simulink model "Simulink_6DoF_RV"  (R2021b)
settings: Solver=ode4  StartTime=0.0  StopTime=T_run  FixedStep=0.01  RelTol=1e-3
values from neighbouring files (symbols this model uses):
  alpha = 5    [MAIN_6DoF_RV.m]    (also in Simulatore_script_gruppo6.m)
  beta = 10    [MAIN_6DoF_RV.m]    (also in Simulatore_script_gruppo6.m)
  control = 2    [MAIN_6DoF_RV.m]    (also in Simulatore_script_gruppo6.m)
  den_pos = [Tm_pos 1]    [MAIN_6DoF_RV.m]    (also in Simulatore_script_gruppo6.m)
  dt_Fx1_PH1 = (1+dtx_PH1_corr)*dt_Fx1_PH1id    (= 48.314973357)    [MAIN_6DoF_RV.m]    (also in Simulatore_script_gruppo6.m)
  Dt_var = 0.1    [MAIN_6DoF_RV.m]    (also in Simulatore_script_gruppo6.m)
  dtz_PH2_corr = 0.28    [MAIN_6DoF_RV.m]    (also in Simulatore_script_gruppo6.m)
  epsilon = 1e-3    (= 0.001)    [MAIN_6DoF_RV.m]    (also in Simulatore_script_gruppo6.m)
  epsilon_FA = 0.005    [MAIN_6DoF_RV.m]    (also in Simulatore_script_gruppo6.m)
  F_D = 1/2*rho*CD*A*vc^2    [MAIN_6DoF_RV.m]    (also in Simulatore_script_gruppo6.m)
  fa_control = 2    [MAIN_6DoF_RV.m]    (also in Simulatore_script_gruppo6.m)
  FJ2_r4 = -mc*(3*J2*mu*r_E^2)/2    (= -1.15338103268e+24)    [MAIN_6DoF_RV.m]    (also in Simulatore_script_gruppo6.m)
  Fx_PH1id = Tmax    (= 1)    [MAIN_6DoF_RV.m]    (also in Simulatore_script_gruppo6.m)
  Fz_PH2id = Tmax    (= 1)    [MAIN_6DoF_RV.m]    (also in Simulatore_script_gruppo6.m)
  I = [Jx  0   0 ... (first row only)    [MAIN_6DoF_RV.m]    (also in Simulatore_script_gruppo6.m)
  Id = eye(3)    [MAIN_6DoF_RV.m]    (also in Simulatore_script_gruppo6.m)
  invI = inv(I)    [MAIN_6DoF_RV.m]    (also in Simulatore_script_gruppo6.m)
  K_d = diag([d1,d2,d3])    [MAIN_6DoF_RV.m]    (also in Simulatore_script_gruppo6.m)
  lambda = 0.06    [MAIN_6DoF_RV.m]    (also in Simulatore_script_gruppo6.m)
  lambda_FA = 0.07    [MAIN_6DoF_RV.m]    (also in Simulatore_script_gruppo6.m)
  mc = 43.8    [MAIN_6DoF_RV.m]    (also in Simulatore_script_gruppo6.m)
  mu = 3.986012*10^14    (= 398601200000000)    [MAIN_6DoF_RV.m]    (also in Simulatore_script_gruppo6.m)
  num_pos = Km_pos    (= 4)    [MAIN_6DoF_RV.m]    (also in Simulatore_script_gruppo6.m)
  omega = (mu/r_t^3)^0.5    (= 0.00113136572666)    [MAIN_6DoF_RV.m]    (also in Simulatore_script_gruppo6.m)
  omega_0 = [0 0 0]    [MAIN_6DoF_RV.m]    (also in Simulatore_script_gruppo6.m)
  q0_0 = 0.5    [MAIN_6DoF_RV.m]    (also in Simulatore_script_gruppo6.m)
  q0_des = quat0_PH3(1)    [MAIN_6DoF_RV.m]    (also in Simulatore_script_gruppo6.m)
  qv_0 = [0.5 0.5 0.5]    [MAIN_6DoF_RV.m]    (also in Simulatore_script_gruppo6.m)
  r0 = [Xo Yo Zo]    [MAIN_6DoF_RV.m]    (also in Simulatore_script_gruppo6.m)
  r0_p1Id = [x0_PH1, y0_PH1, z0_PH1]    [MAIN_6DoF_RV.m]    (also in Simulatore_script_gruppo6.m)
  r0_p3Id = [x0_PH3 y0_PH3 z0_PH3]    [MAIN_6DoF_RV.m]    (also in Simulatore_script_gruppo6.m)
  r_des_fa = [xf yf zf]    [MAIN_6DoF_RV.m]    (also in Simulatore_script_gruppo6.m)
  r_t = r_E + height    (= 6778145)    [MAIN_6DoF_RV.m]    (also in Simulatore_script_gruppo6.m)
  t_acc_fa = (1+dtx_PH3_corr)*t_acc_fa_id    [MAIN_6DoF_RV.m]    (also in Simulatore_script_gruppo6.m)
  tau_RW = 0.25    [MAIN_6DoF_RV.m]    (also in Simulatore_script_gruppo6.m)
  Tmax = n*Fthr    (= 1)    [MAIN_6DoF_RV.m]    (also in Simulatore_script_gruppo6.m)
  U_max = 0.25    [MAIN_6DoF_RV.m]    (also in Simulatore_script_gruppo6.m)
  U_max_RW = 1e-3    (= 0.001)    [MAIN_6DoF_RV.m]    (also in Simulatore_script_gruppo6.m)
  U_off_pos = 0.60*U_on_pos    (= 0.6)    [MAIN_6DoF_RV.m]    (also in Simulatore_script_gruppo6.m)
  U_on_pos = 1    [MAIN_6DoF_RV.m]    (also in Simulatore_script_gruppo6.m)
  v0 = [Vxo Vyo Vzo]    [MAIN_6DoF_RV.m]    (also in Simulatore_script_gruppo6.m)
  v_des_fa = [vxf vyf vzf]    [MAIN_6DoF_RV.m]    (also in Simulatore_script_gruppo6.m)
  Vx_max = 0.15    [MAIN_6DoF_RV.m]    (also in Simulatore_script_gruppo6.m)
  x0_PH2 = -3000    [MAIN_6DoF_RV.m]    (also in Simulatore_script_gruppo6.m)
  x0_PH3 = -500    [MAIN_6DoF_RV.m]    (also in Simulatore_script_gruppo6.m)
  x_start_dec = r_des_fa(1)-(v_des_fa(1)^2-(Vx_max*(1+dtx_PH3_corr))^2)/(2*(Fx_dec/mc))    [MAIN_6DoF_RV.m]    (also in Simulatore_script_gruppo6.m)
  xf = -2    [MAIN_6DoF_RV.m]    (also in Simulatore_script_gruppo6.m)
  Z0_RW = [sqrt(3)/2    0           -sqrt(3)/2  0 ... (first row only)    [MAIN_6DoF_RV.m]    (also in Simulatore_script_gruppo6.m)
  z_start_Fx2_PH1id = 0.5*(DVx2*(1+dtx_PH1_corr))^2/(Fx_PH1id/mc)    (= 26.6476786585)    [MAIN_6DoF_RV.m]    (also in Simulatore_script_gruppo6.m)
  z_start_Fz2_PH2id = 0.5*(DVz2*(1+dtz_PH2_corr))^2/(Fz_PH2id/mc)    [MAIN_6DoF_RV.m]    (also in Simulatore_script_gruppo6.m)
  Zinv = pinv(Z0_RW)    [MAIN_6DoF_RV.m]    (also in Simulatore_script_gruppo6.m)
libraries: vrlib x3, robotcorelib x1
(part 1 of 2)
settings Model: SimulationMode=rapid-accelerator  Creator=Asus  LastModifiedBy=Asus
settings SolverCC: AlgebraicLoopSolver=TrustRegion
settings DebuggingCC: ArithmeticOperatorsInVariantConditions=warning
settings SFSimCC: CustomCodeUndefinedFunction=UseInterfaceOnly

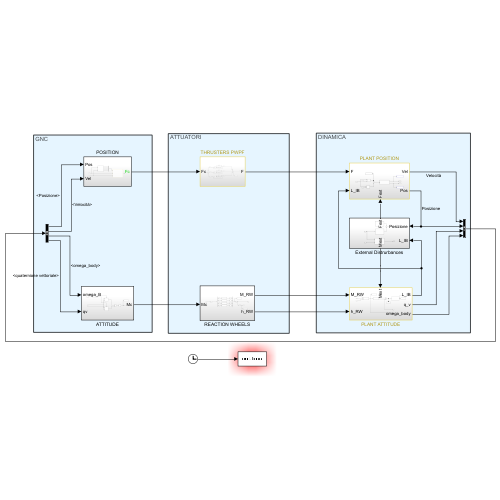
[thumbnail: Simulink's stored preview of the top-level diagram]
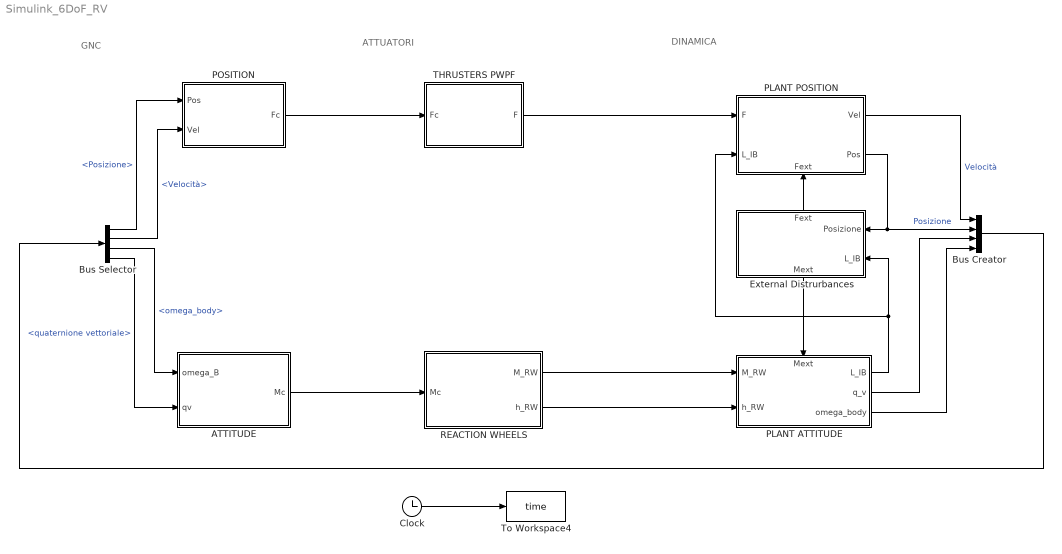
== system Simulink_6DoF_RV ==
  note: DINAMICA
  note: ATTUATORI
  note: GNC
  ATTITUDE : Subsystem  SystemSampleTime=0.02
  Bus Creator : BusCreator  Inputs=4
  Bus Selector : BusSelector  OutputSignals=Posizione,Velocità,omega_body,quaternione vettoriale
  Clock : Clock
  External Distrurbances : Subsystem
      settings: PortSchema="{\"entries\":[{\"content\":{\"sides\":[{\"content\":{\"connectorIds\":[]},\"type\":\"ConnectorPlacement.EquallySpacedRectSide\",\"uuid\":\"40a47393-8969-4a4a-bb19-fe76317a4dc1\"},{\"content\":{\"connectorIds\":[\"In1\",\"In2\"],\"side\":\"RIGHT\"},\"type\":\"ConnectorPlacement.EquallySpacedRectSide\",\"uuid\":\"517d6888-1d4e-40fb-9a61-dcbe45465223\"},{\"content\":{\"connectorIds\":[\"Out2\"],\"side\":\"TOP\"},\"type\":\"ConnectorPlacement.EquallySpacedRectSide\",\"uuid\":\"885891b7-149a-48f0-ba9b-916a7b55094e\"},{\"content\":{\"connectorIds\":[\"Out1\"],\"side\":\"BOTTOM\"},\"type\":\"ConnectorPlacement.EquallySpacedRectSide\",\"uuid\":\"c8000deb-5487-4091-9eab-42d91257081e\"}]},\"type\":\"ConnectorPlacement.EquallySpacedConnector\",\"uuid\":\"af16e5ba-db8c-4edd-a4d6-30205250b632\"}],\"packageUris\":[\"http://schema.mathworks.com/mf0/Connector/R2020b\"],\"version\":\"1.0\"}"
  PLANT ATTITUDE : Subsystem
      settings: PortSchema="{\"entries\":[{\"content\":{\"sides\":[{\"content\":{\"connectorIds\":[\"In1\",\"In2\"]},\"type\":\"ConnectorPlacement.EquallySpacedRectSide\",\"uuid\":\"5bd07662-f93f-4a51-a4b7-c766d18c6c52\"},{\"content\":{\"connectorIds\":[\"Out1\",\"Out2\",\"Out3\"],\"side\":\"RIGHT\"},\"type\":\"ConnectorPlacement.EquallySpacedRectSide\",\"uuid\":\"400ce1e4-a5e5-4d4b-bb84-f2deb9eca011\"},{\"content\":{\"connectorIds\":[\"In3\"],\"side\":\"TOP\"},\"type\":\"ConnectorPlacement.EquallySpacedRectSide\",\"uuid\":\"a16ccc55-2fa1-4b33-bfe9-424ec0136aee\"}]},\"type\":\"ConnectorPlacement.EquallySpacedConnector\",\"uuid\":\"0051f69f-69f8-4575-b5c3-4b5124977914\"}],\"packageUris\":[\"http://schema.mathworks.com/mf0/Connector/R2020b\"],\"version\":\"1.0\"}"
  PLANT POSITION : Subsystem
      settings: PortSchema="{\"entries\":[{\"content\":{\"sides\":[{\"content\":{\"connectorIds\":[\"In1\",\"In2\"]},\"type\":\"ConnectorPlacement.EquallySpacedRectSide\",\"uuid\":\"6f851545-3e44-41e1-9040-e1da3530ae0f\"},{\"content\":{\"connectorIds\":[\"Out1\",\"Out2\"],\"side\":\"RIGHT\"},\"type\":\"ConnectorPlacement.EquallySpacedRectSide\",\"uuid\":\"a0bf2e2b-c069-45ff-9cba-5c6c5f5dd88c\"},{\"content\":{\"connectorIds\":[],\"side\":\"TOP\"},\"type\":\"ConnectorPlacement.EquallySpacedRectSide\",\"uuid\":\"79f05063-7ba4-40b0-bcbd-aeb89fa83470\"},{\"content\":{\"connectorIds\":[\"In3\"],\"side\":\"BOTTOM\"},\"type\":\"ConnectorPlacement.EquallySpacedRectSide\",\"uuid\":\"12fcf113-d807-4585-8c70-f8ca37fce548\"}]},\"type\":\"ConnectorPlacement.EquallySpacedConnector\",\"uuid\":\"de90291e-fe15-4172-840f-0b421646e685\"}],\"packageUris\":[\"http://schema.mathworks.com/mf0/Connector/R2020b\"],\"version\":\"1.0\"}"
  POSITION : Subsystem  SystemSampleTime=0.01
      settings: MinAlgLoopOccurrences=on
  REACTION WHEELS : Subsystem
  THRUSTERS PWPF : Subsystem
  To Workspace4 : ToWorkspace  VariableName=time  SampleTime=Dt_var
  wires:
  Clock/1 -> To Workspace4/1
  PLANT POSITION/2(Pos) -> External Distrurbances/1(Posizione), Bus Creator/2  "Posizione"
  PLANT POSITION/1(Vel) -> Bus Creator/1  "Velocità"
  REACTION WHEELS/2(h_RW) -> PLANT ATTITUDE/2(h_RW)
  REACTION WHEELS/1(M_RW) -> PLANT ATTITUDE/1(M_RW)
  PLANT ATTITUDE/2(q_v) -> Bus Creator/3
  PLANT ATTITUDE/3(omega_body) -> Bus Creator/4
  ATTITUDE/1(Mc) -> REACTION WHEELS/1(Mc)
  Bus Selector/3 -> ATTITUDE/1(omega_B)  "<omega_body>"
  Bus Selector/4 -> ATTITUDE/2(qv)  "<quaternione vettoriale>"
  PLANT ATTITUDE/1(L_IB) -> External Distrurbances/2(L_IB), PLANT POSITION/2(L_IB)
  Bus Selector/1 -> POSITION/1(Pos)  "<Posizione>"
  Bus Selector/2 -> POSITION/2(Vel)  "<Velocità>"
  External Distrurbances/1(Mext) -> PLANT ATTITUDE/3(Mext)
  POSITION/1(Fc) -> THRUSTERS PWPF/1(Fc)
  Bus Creator/1 -> Bus Selector/1
  THRUSTERS PWPF/1(F) -> PLANT POSITION/1(F)
  External Distrurbances/2(Fext) -> PLANT POSITION/3(Fext)

== system Simulink_6DoF_RV/ATTITUDE ==
  omega_B : Inport
  qv : Inport  Port=2
  Constant : Constant  Value=control
  Merge : Merge
  PD 4 : Subsystem  TreatAsAtomicUnit=on
  Rate Transition : RateTransition  OutPortSampleTime=0.02
  SMC : Subsystem  TreatAsAtomicUnit=on
  Switch Case : SwitchCase  CaseConditions={2,1}  ShowDefaultCase=off
  To Workspace2 : ToWorkspace  VariableName=Mc  SampleTime=Dt_var
  Mc : Outport
  wires:
  Merge/1 -> Rate Transition/1
  Switch Case/2 -> PD 4/Action
  PD 4/1(Mc) -> Merge/2
  Constant/1 -> Switch Case/1
  omega_B/1 -> SMC/1("omega_B "), PD 4/1(omega_B)  "omega_body"
  SMC/1(Mc) -> Merge/1
  Switch Case/1 -> SMC/Action
  qv/1 -> PD 4/2(qv), SMC/2(qv)  "quaternione vettoriale"
  Rate Transition/1 -> To Workspace2/1, Mc/1

== system Simulink_6DoF_RV/External Distrurbances ==
  Posizione : Inport
  L_IB : Inport  Port=2
  Drag : Subsystem
  Gravity Gradient : Subsystem
  J2 : Subsystem
  Sum : Sum
  Mext : Outport
  Fext : Outport  Port=2
  wires:
  Drag/1(Fa) -> Sum/1
  Sum/1 -> Fext/1
  J2/1(Fj2) -> Sum/2
  Gravity Gradient/1(Mgg) -> Mext/1
  Posizione/1 -> Gravity Gradient/1(Posizione1), J2/1(Posizione)
  L_IB/1 -> Gravity Gradient/2(L_IB)

== system Simulink_6DoF_RV/PLANT ATTITUDE ==
  M_RW : Inport
  h_RW : Inport  Port=2
  Mext : Inport  Port=3
  Coordinate Transformation Conversion : robotcorelib/Coordinate Transformation Conversion  InputRepresentation=Quaternion  InputEulerSequence=ZYX  ShowTrVecInputPort=on  OutputRepresentation=Rotation Matrix  OutputEulerSequence=ZYX  ShowTrVecOutputPort=on  SimulateUsing=Interpreted execution
      settings: SourceProductBaseCode=NV,RO,RR,UV
  Eq. eulero : Subsystem
  Mux : Mux  Inputs=2
  To Workspace : ToWorkspace  VariableName=omega_B  SampleTime=Dt_var
  To Workspace1 : ToWorkspace  VariableName=q  SampleTime=Dt_var
  To Workspace5 : ToWorkspace  VariableName=L  SampleTime=Dt_var
  quaternioni : Subsystem
  L_IB : Outport
  q_v : Outport  Port=2
  omega_body : Outport  Port=3
  wires:
  quaternioni/1(q0) -> Mux/1
  Eq. eulero/1(omega_B) -> To Workspace/1, omega_body/1, quaternioni/1(omega_B)  "omega_body"
  Mux/1 -> Coordinate Transformation Conversion/1, To Workspace1/1
  M_RW/1 -> Eq. eulero/3(M_RW)
  h_RW/1 -> Eq. eulero/2(h_RW)
  Coordinate Transformation Conversion/1 -> L_IB/1, To Workspace5/1
  quaternioni/2(qv) -> q_v/1, Mux/2  "quaternione vettoriale"
  Mext/1 -> Eq. eulero/1(M)

== system Simulink_6DoF_RV/PLANT POSITION ==
  F : Inport
  L_IB : Inport  Port=2
  Fext : Inport  Port=3
  HILL eqs : Subsystem
  Matrix Multiply : Product  Multiplication=Matrix(*)
  Matrix Multiply1 : Product  Multiplication=Matrix(*)
  Sum3 : Sum
  To Workspace1 : ToWorkspace  VariableName=Pos  SampleTime=Dt_var
  To Workspace2 : ToWorkspace  VariableName=Vel  SampleTime=Dt_var
  To Workspace3 : ToWorkspace  VariableName=F_LVLH  SampleTime=Dt_var
  Vel : Outport
  Pos : Outport  Port=2
  wires:
  F/1 -> Matrix Multiply1/2
  L_IB/1 -> Matrix Multiply/1, Matrix Multiply1/1
  Matrix Multiply1/1 -> To Workspace3/1, Sum3/1
  Matrix Multiply/1 -> Sum3/2
  Fext/1 -> Matrix Multiply/2
  HILL eqs/2(Out2) -> To Workspace2/1, Vel/1
  Sum3/1 -> HILL eqs/1(In1)
  HILL eqs/1(Pos) -> To Workspace1/1, Pos/1

== system Simulink_6DoF_RV/POSITION ==
  Pos : Inport
  Vel : Inport  Port=2
  Bus Creator : BusCreator  Inputs=5
  Maneuvers : Subsystem
  Position and Guidance : Subsystem
  Fc : Outport
  wires:
  Vel/1 -> Position and Guidance/3(Vel), Maneuvers/2(Vel)
  Pos/1 -> Position and Guidance/2(Pos), Maneuvers/1(Pos)
  Position and Guidance/1(Fc) -> Fc/1
  Maneuvers/1(Phase number) -> Bus Creator/1  "phase number"
  Maneuvers/2(off_PH1.1) -> Bus Creator/2  "off_PH1:1"
  Maneuvers/3(off_PH1.2) -> Bus Creator/3  "off_PH1:2"
  Maneuvers/4(off_PH2.1) -> Bus Creator/4  "off_PH2:1"
  Maneuvers/5(off_PH2.2) -> Bus Creator/5  "off_PH2:2"
  Bus Creator/1 -> Position and Guidance/1(Phase)

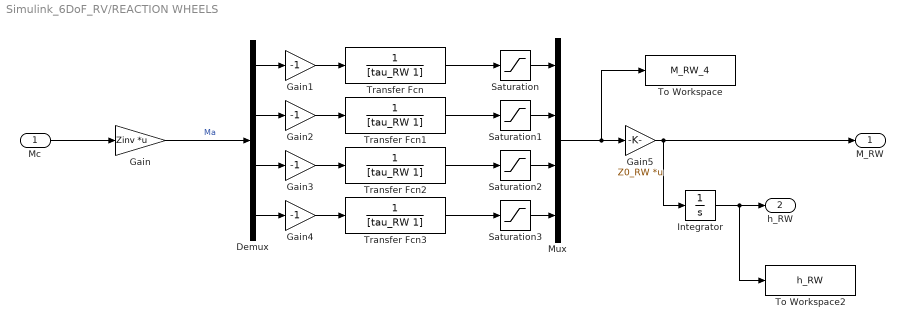
== system Simulink_6DoF_RV/REACTION WHEELS ==
  Mc : Inport
  Demux : Demux
  Gain : Gain  Gain=Zinv  Multiplication=Matrix(K*u)
  Gain{1..4} (4 alike) : Gain  Gain=-1
  Gain5 : Gain  Gain=Z0_RW  Multiplication=Matrix(K*u)
  Integrator : Integrator
  Mux : Mux
  Saturation{,1..3} (4 alike) : Saturate  UpperLimit=U_max_RW  LowerLimit=-U_max_RW
  To Workspace : ToWorkspace  VariableName=M_RW_4  SampleTime=Dt_var
  To Workspace2 : ToWorkspace  VariableName=h_RW  SampleTime=Dt_var
  Transfer Fcn{,1..3} (4 alike) : TransferFcn  Denominator=[tau_RW 1]
  M_RW : Outport
  h_RW : Outport  Port=2
  wires:
  Demux/4 -> Gain4/1
  Mc/1 -> Gain/1
  Demux/1 -> Gain1/1
  Transfer Fcn2/1 -> Saturation2/1
  Gain3/1 -> Transfer Fcn2/1
  Gain/1 -> Demux/1  "Ma"
  Saturation/1 -> Mux/1
  Gain5/1 -> M_RW/1, Integrator/1
  Gain4/1 -> Transfer Fcn3/1
  Transfer Fcn3/1 -> Saturation3/1
  Saturation3/1 -> Mux/4
  Transfer Fcn1/1 -> Saturation1/1
  Gain2/1 -> Transfer Fcn1/1
  Transfer Fcn/1 -> Saturation/1
  Saturation2/1 -> Mux/3
  Demux/3 -> Gain3/1
  Gain1/1 -> Transfer Fcn/1
  Integrator/1 -> To Workspace2/1, h_RW/1
  Mux/1 -> To Workspace/1, Gain5/1
  Demux/2 -> Gain2/1
  Saturation1/1 -> Mux/2

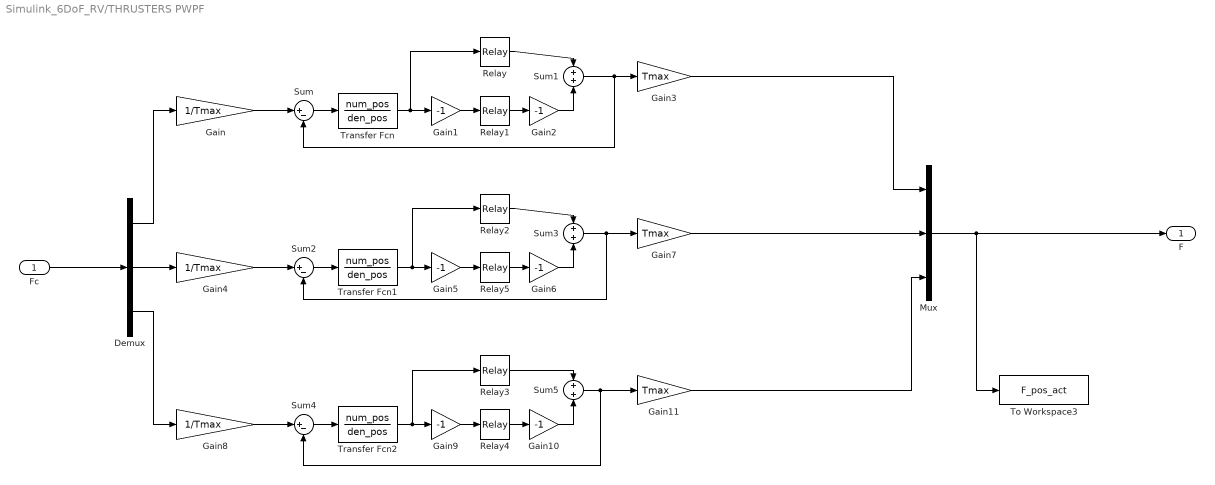
== system Simulink_6DoF_RV/THRUSTERS PWPF ==
  Fc : Inport
  Demux : Demux  Outputs=3
  Gain : Gain  Gain=1/Tmax
  Gain{1..2,5..6,9..10} (6 alike) : Gain  Gain=-1
  Gain11 : Gain  Gain=Tmax
  Gain3 : Gain  Gain=Tmax
  Gain4 : Gain  Gain=1/Tmax
  Gain7 : Gain  Gain=Tmax
  Gain8 : Gain  Gain=1/Tmax
  Mux : Mux  Inputs=3
  Relay{,1..5} (6 alike) : Relay  OnSwitchValue=U_on_pos  OffSwitchValue=U_off_pos
  Sum : Sum  Inputs=|+-
  Sum1 : Sum  Inputs=+|+
  Sum2 : Sum  Inputs=|+-
  Sum3 : Sum  Inputs=+|+
  Sum4 : Sum  Inputs=|+-
  Sum5 : Sum  Inputs=+|+
  To Workspace3 : ToWorkspace  VariableName=F_pos_act  SampleTime=Dt_var
  Transfer Fcn : TransferFcn  Numerator=num_pos  Denominator=den_pos
  Transfer Fcn1 : TransferFcn  Numerator=num_pos  Denominator=den_pos
  Transfer Fcn2 : TransferFcn  Numerator=num_pos  Denominator=den_pos
  F : Outport
  wires:
  Demux/1 -> Gain/1
  Gain/1 -> Sum/1
  Gain1/1 -> Relay1/1
  Relay1/1 -> Gain2/1
  Relay/1 -> Sum1/1
  Gain2/1 -> Sum1/2
  Sum1/1 -> Gain3/1, Sum/2
  Gain3/1 -> Mux/1
  Transfer Fcn/1 -> Gain1/1, Relay/1
  Sum/1 -> Transfer Fcn/1
  Mux/1 -> F/1, To Workspace3/1
  Transfer Fcn1/1 -> Relay2/1, Gain5/1
  Relay5/1 -> Gain6/1
  Sum3/1 -> Sum2/2, Gain7/1
  Relay2/1 -> Sum3/1
  Gain7/1 -> Mux/2
  Gain4/1 -> Sum2/1
  Demux/2 -> Gain4/1
  Sum2/1 -> Transfer Fcn1/1
  Gain6/1 -> Sum3/2
  Gain5/1 -> Relay5/1
  Gain10/1 -> Sum5/2
  Gain11/1 -> Mux/3
  Sum4/1 -> Transfer Fcn2/1
  Sum5/1 -> Sum4/2, Gain11/1
  Relay4/1 -> Gain10/1
  Transfer Fcn2/1 -> Relay3/1, Gain9/1
  Gain9/1 -> Relay4/1
  Relay3/1 -> Sum5/1
  Gain8/1 -> Sum4/1
  Demux/3 -> Gain8/1
  Fc/1 -> Demux/1

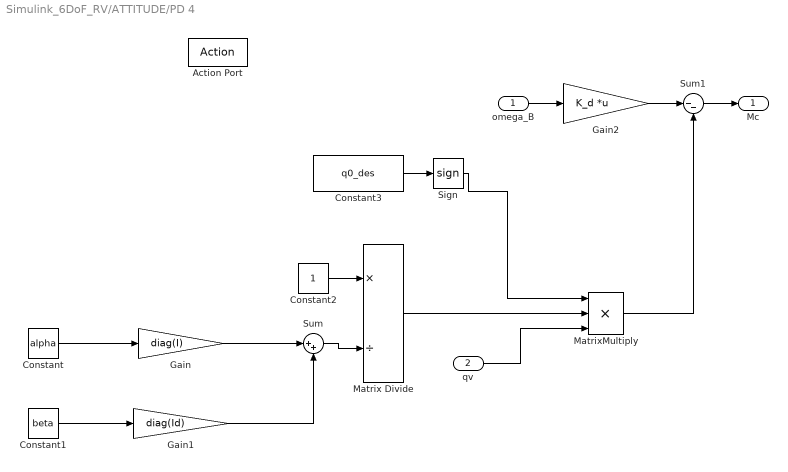
== system Simulink_6DoF_RV/ATTITUDE/PD 4 ==
  omega_B : Inport
  qv : Inport  Port=2
  Action Port : ActionPort  ActionPortLabel=case [ 1 ]:
  Constant : Constant  Value=alpha
  Constant1 : Constant  Value=beta
  Constant2 : Constant
  Constant3 : Constant  Value=q0_des
  Gain : Gain  Gain=diag(I)
  Gain1 : Gain  Gain=diag(Id)
  Gain2 : Gain  Gain=K_d  Multiplication=Matrix(K*u)
  Matrix Divide : Product  Inputs=*/
  MatrixMultiply : Product  Inputs=3
  Sign : Signum
  Sum : Sum  Inputs=|++
  Sum1 : Sum  Inputs=|--
  Mc : Outport
  wires:
  Constant2/1 -> Matrix Divide/1
  qv/1 -> MatrixMultiply/3
  Sum1/1 -> Mc/1
  Matrix Divide/1 -> MatrixMultiply/2
  Constant3/1 -> Sign/1
  MatrixMultiply/1 -> Sum1/2
  Constant1/1 -> Gain1/1
  omega_B/1 -> Gain2/1
  Gain/1 -> Sum/1
  Sum/1 -> Matrix Divide/2
  Constant/1 -> Gain/1
  Gain1/1 -> Sum/2
  Gain2/1 -> Sum1/1
  Sign/1 -> MatrixMultiply/1

== system Simulink_6DoF_RV/ATTITUDE/SMC ==
  "omega_B " : Inport
  qv : Inport  Port=2
  Action Port : ActionPort  ActionPortLabel=case [ 2 ]:
  Constant : Constant  Value="[U_max  U_max_RW]"
  Constant1 : Constant  Value=[lambda, epsilon]
  Constant2 : Constant  Value=control
  MATLAB Function : MATLAB Function  TreatAsAtomicUnit=on
  Mc : Outport
  wires:
  "omega_B "/1 -> MATLAB Function/1(omega_B)
  qv/1 -> MATLAB Function/2(qv)
  Constant1/1 -> MATLAB Function/4(ctrl_var)
  Constant/1 -> MATLAB Function/3(max)
  MATLAB Function/1(y) -> Mc/1
  Constant2/1 -> MATLAB Function/5(control)

== system Simulink_6DoF_RV/External Distrurbances/Drag ==
  Constant : Constant  Value=F_D
  Gain : Gain  Gain=[-1 0 0]
  Fa : Outport
  wires:
  Gain/1 -> Fa/1
  Constant/1 -> Gain/1

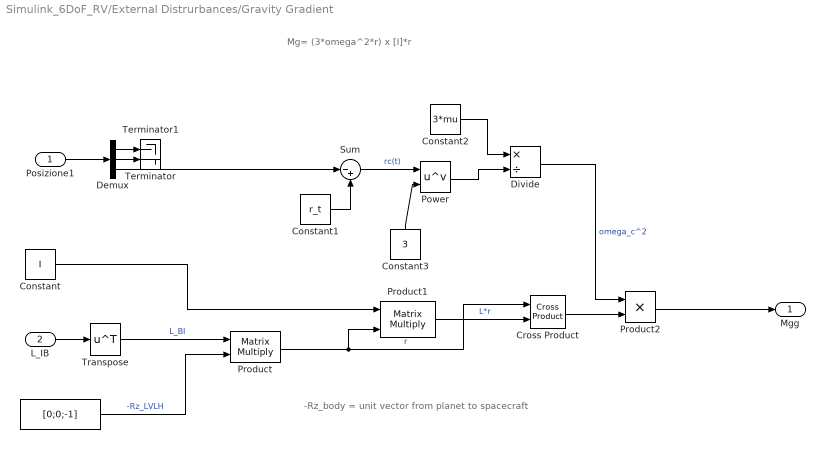
== system Simulink_6DoF_RV/External Distrurbances/Gravity Gradient ==
  note: -Rz_body = unit vector from planet to spacecraft
  note: Mg= (3*omega^2*r) x [I]*r
  Posizione1 : Inport
  L_IB : Inport  Port=2
  " " : Constant  Value=[0;0;-1]
  Constant : Constant  Value=I
  Constant1 : Constant  Value=r_t
  Constant2 : Constant  Value=3*mu
  Constant3 : Constant  Value=3
  Cross Product : vrlib/Utilities/Cross Product
  Demux : Demux  Outputs=3
  Divide : Product  Inputs=*/
  Power : Math  Operator=pow  SaturateOnIntegerOverflow=on
  Product : Product  Multiplication=Matrix(*)
  Product1 : Product  Multiplication=Matrix(*)
  Product2 : Product
  Sum : Sum  Inputs=|-+
  Terminator : Terminator
  Terminator1 : Terminator
  Transpose : Math  Operator=transpose  SaturateOnIntegerOverflow=on
  Mgg : Outport
  wires:
  " "/1 -> Product/2  "-Rz_LVLH"
  Product/1 -> Cross Product/1, Product1/2  "r"
  Constant/1 -> Product1/1
  Product1/1 -> Cross Product/2  "L*r"
  Cross Product/1 -> Product2/2
  Product2/1 -> Mgg/1
  L_IB/1 -> Transpose/1
  Transpose/1 -> Product/1  "L_BI"
  Posizione1/1 -> Demux/1
  Demux/3 -> Sum/1
  Demux/2 -> Terminator/1
  Demux/1 -> Terminator1/1
  Constant1/1 -> Sum/2
  Constant2/1 -> Divide/1
  Divide/1 -> Product2/1  "omega_c^2"
  Sum/1 -> Power/1  "rc(t)"
  Power/1 -> Divide/2
  Constant3/1 -> Power/2

== system Simulink_6DoF_RV/External Distrurbances/J2 ==
  Posizione : Inport
  Constant : Constant  Value=FJ2_r4
  Constant1 : Constant  Value=r_t
  Constant3 : Constant  Value=4
  Demux : Demux  Outputs=3
  Divide : Product  Inputs=*/
  Gain : Gain  Gain=[1 1 1]
  Power : Math  Operator=pow  SaturateOnIntegerOverflow=on
  Sum : Sum  Inputs=-|+
  Terminator : Terminator
  Terminator1 : Terminator
  Fj2 : Outport
  wires:
  Gain/1 -> Fj2/1
  Posizione/1 -> Demux/1
  Demux/2 -> Terminator/1
  Demux/1 -> Terminator1/1
  Constant1/1 -> Sum/2
  Demux/3 -> Sum/1
  Sum/1 -> Power/1  "rc(t)"
  Constant3/1 -> Power/2
  Power/1 -> Divide/2  "r^4"
  Constant/1 -> Divide/1  "Fj2*r^4"
  Divide/1 -> Gain/1

== system Simulink_6DoF_RV/PLANT ATTITUDE/Eq. eulero ==
  note: omega_B x I*omega_B
  note: omega_dot_B=inv(I)*(M-(omega_B x I*omega_B))
  note: omega_dot_B
  M : Inport
  h_RW : Inport  Port=2
  M_RW : Inport  Port=3
  Cross Product : vrlib/Utilities/Cross Product
  Gain : Gain  Gain=invI  Multiplication=Matrix(K*u)
  Integrator : Integrator  InitialCondition=omega_0
  Subtract : Sum  Inputs=+--
  Sum : Sum  Inputs=|++
  matrice di inerzia : Gain  Gain=I  Multiplication=Matrix(K*u)
  omega_B : Outport
  wires:
  Cross Product/1 -> Subtract/3
  M_RW/1 -> Subtract/2
  matrice di inerzia/1 -> Sum/1  "I x oemga_B"
  Subtract/1 -> Gain/1
  Gain/1 -> Integrator/1
  Integrator/1 -> Cross Product/1, matrice di inerzia/1, omega_B/1  "omega_B"
  h_RW/1 -> Sum/2
  Sum/1 -> Cross Product/2
  M/1 -> Subtract/1

== system Simulink_6DoF_RV/PLANT ATTITUDE/quaternioni ==
  note: qv
  note: omega_B
  note: qv_dot
  note: q0_dot
  note: omega_B X qv
  note: q0*omega_B
  omega_B : Inport
  Cross Product1 : vrlib/Utilities/Cross Product
  Dot Product : DotProduct  InputSameDT=on  OutDataTypeStr=Inherit: Inherit via internal rule
  Gain : Gain  Gain=-0.5
  Gain1 : Gain  Gain=0.5
  Integrator : Integrator  InitialCondition=q0_0
  Integrator1 : Integrator  InitialCondition=qv_0
  Product : Product
  Subtract : Sum  Inputs=+-
  q0 : Outport
  qv : Outport  Port=2
  wires:
  omega_B/1 -> Dot Product/2, Cross Product1/1, Product/2
  Dot Product/1 -> Gain/1
  Integrator/1 -> Product/1, q0/1
  Integrator1/1 -> qv/1, Dot Product/1, Cross Product1/2
  Product/1 -> Subtract/1
  Cross Product1/1 -> Subtract/2
  Subtract/1 -> Gain1/1
  Gain1/1 -> Integrator1/1  "1/2*(q0*omega_B-omega_B x qv)"
  Gain/1 -> Integrator/1  "-1/2*omega_B*q"

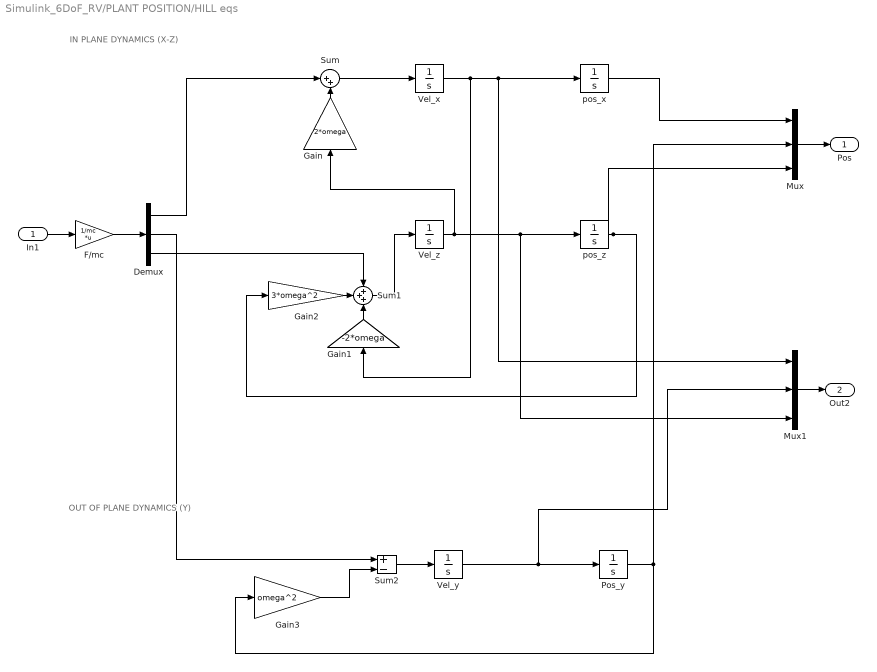
== system Simulink_6DoF_RV/PLANT POSITION/HILL eqs ==
  note: OUT OF PLANE DYNAMICS (Y)
  note: IN PLANE DYNAMICS (X-Z)
  In1 : Inport
  Demux : Demux  Outputs=3
  F/mc : Gain  Gain=1/mc  Multiplication=Matrix(K*u)
  Gain : Gain  Gain=2*omega
  Gain1 : Gain  Gain=-2*omega
  Gain2 : Gain  Gain=3*omega^2
  Gain3 : Gain  Gain=omega^2
  Mux : Mux  Inputs=3
  Mux1 : Mux  Inputs=3
  Pos_y : Integrator  InitialCondition=r0(2)
  Sum : Sum  Inputs=|++
  Sum1 : Sum  Inputs=+++
  Sum2 : Sum  Inputs=+-
  Vel_x : Integrator  InitialCondition=v0(1)
  Vel_y : Integrator  InitialCondition=v0(2)
  Vel_z : Integrator  InitialCondition=v0(3)
  pos_x : Integrator  InitialCondition=r0(1)
  pos_z : Integrator  InitialCondition=r0(3)
  Pos : Outport
  Out2 : Outport  Port=2
  wires:
  In1/1 -> F/mc/1
  Vel_x/1 -> Gain1/1, Mux1/1, pos_x/1
  Vel_z/1 -> pos_z/1, Mux1/3, Gain/1
  Vel_y/1 -> Mux1/2, Pos_y/1
  Sum/1 -> Vel_x/1
  pos_z/1 -> Mux/3, Gain2/1
  Pos_y/1 -> Gain3/1, Mux/2
  Mux/1 -> Pos/1
  Gain1/1 -> Sum1/3
  Demux/2 -> Sum2/1
  Gain3/1 -> Sum2/2
  Sum1/1 -> Vel_z/1
  pos_x/1 -> Mux/1
  Gain2/1 -> Sum1/2
  Gain/1 -> Sum/2
  F/mc/1 -> Demux/1
  Sum2/1 -> Vel_y/1
  Demux/3 -> Sum1/1
  Demux/1 -> Sum/1
  Mux1/1 -> Out2/1

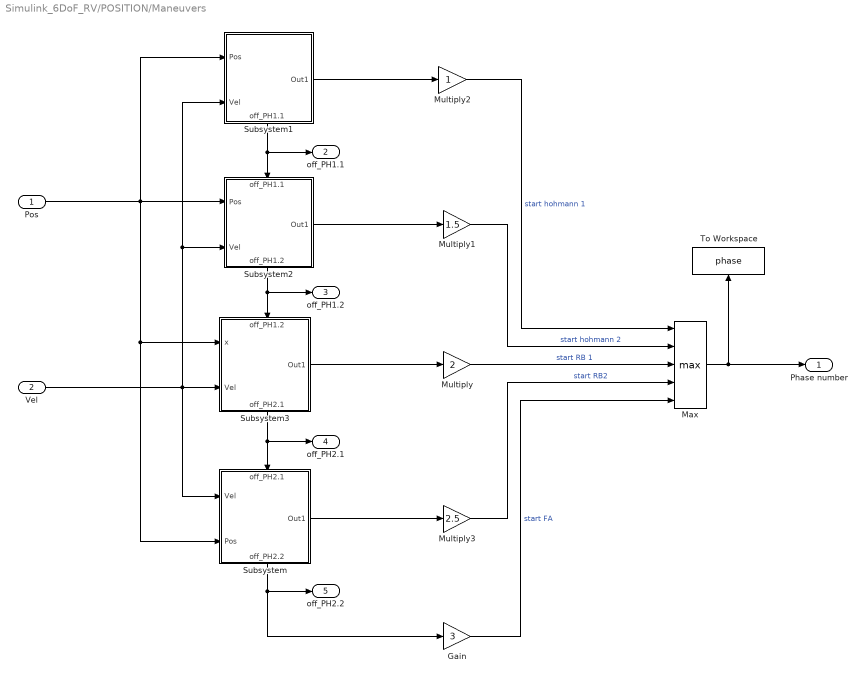
== system Simulink_6DoF_RV/POSITION/Maneuvers ==
  Pos : Inport
  Vel : Inport  Port=2
  Gain : Gain  Gain=3
  Max : MinMax  Function=max  Inputs=5
  Multiply : Gain  Gain=2
  Multiply1 : Gain  Gain=1.5
  Multiply2 : Gain
  Multiply3 : Gain  Gain=2.5
  Subsystem : Subsystem
      settings: PortSchema="{\"entries\":[{\"content\":{\"sides\":[{\"content\":{\"connectorIds\":[\"In1\",\"In2\"]},\"type\":\"ConnectorPlacement.EquallySpacedRectSide\",\"uuid\":\"42e6cdd5-7474-45c6-b8eb-e025beecc22a\"},{\"content\":{\"connectorIds\":[\"Out1\"],\"side\":\"RIGHT\"},\"type\":\"ConnectorPlacement.EquallySpacedRectSide\",\"uuid\":\"d04b3acc-746b-4d28-b374-523a35068b99\"},{\"content\":{\"connectorIds\":[\"In3\"],\"side\":\"TOP\"},\"type\":\"ConnectorPlacement.EquallySpacedRectSide\",\"uuid\":\"0ccae201-7e6b-49e9-bb7a-81c5ae8807ce\"},{\"content\":{\"connectorIds\":[\"Out2\"],\"side\":\"BOTTOM\"},\"type\":\"ConnectorPlacement.EquallySpacedRectSide\",\"uuid\":\"15b38ca0-940d-446d-b70c-188bcbd58912\"}]},\"type\":\"ConnectorPlacement.EquallySpacedConnector\",\"uuid\":\"28dc70bb-edf9-4fda-99b8-5e22fc27861c\"}],\"packageUris\":[\"http://schema.mathworks.com/mf0/Connector/R2020b\"],\"version\":\"1.0\"}"
  Subsystem1 : Subsystem
      settings: PortSchema="{\"entries\":[{\"content\":{\"sides\":[{\"content\":{\"connectorIds\":[\"In1\",\"In2\"]},\"type\":\"ConnectorPlacement.EquallySpacedRectSide\",\"uuid\":\"bf2be483-9c93-43e4-ad10-21dd0c2d669b\"},{\"content\":{\"connectorIds\":[\"Out1\"],\"side\":\"RIGHT\"},\"type\":\"ConnectorPlacement.EquallySpacedRectSide\",\"uuid\":\"8b0ec817-c262-4d55-ab19-261c35555a12\"},{\"content\":{\"connectorIds\":[],\"side\":\"TOP\"},\"type\":\"ConnectorPlacement.EquallySpacedRectSide\",\"uuid\":\"e7d32004-ba09-4bb0-95e5-c1dfa2570e33\"},{\"content\":{\"connectorIds\":[\"Out2\"],\"side\":\"BOTTOM\"},\"type\":\"ConnectorPlacement.EquallySpacedRectSide\",\"uuid\":\"10fbe47b-93fc-47d8-8a40-4f0fc6a502c4\"}]},\"type\":\"ConnectorPlacement.EquallySpacedConnector\",\"uuid\":\"976ec777-b725-4065-a722-c0a3013af977\"}],\"packageUris\":[\"http://schema.mathworks.com/mf0/Connector/R2020b\"],\"version\":\"1.0\"}"
  Subsystem2 : Subsystem
      settings: PortSchema="{\"entries\":[{\"content\":{\"sides\":[{\"content\":{\"connectorIds\":[\"In1\",\"In2\"]},\"type\":\"ConnectorPlacement.EquallySpacedRectSide\",\"uuid\":\"75acc1de-9d0c-42c0-bc9f-344ebaa8143a\"},{\"content\":{\"connectorIds\":[\"Out1\"],\"side\":\"RIGHT\"},\"type\":\"ConnectorPlacement.EquallySpacedRectSide\",\"uuid\":\"244e9f1a-af67-42e6-b4f5-fe935e0b238b\"},{\"content\":{\"connectorIds\":[\"In3\"],\"side\":\"TOP\"},\"type\":\"ConnectorPlacement.EquallySpacedRectSide\",\"uuid\":\"35b5019e-052c-4aa9-b1d7-69ed51f6e4fd\"},{\"content\":{\"connectorIds\":[\"Out2\"],\"side\":\"BOTTOM\"},\"type\":\"ConnectorPlacement.EquallySpacedRectSide\",\"uuid\":\"f42c5389-0220-4180-89cd-e1b6ef8bffa7\"}]},\"type\":\"ConnectorPlacement.EquallySpacedConnector\",\"uuid\":\"40205923-0101-4348-a820-9ef4af731524\"}],\"packageUris\":[\"http://schema.mathworks.com/mf0/Connector/R2020b\"],\"version\":\"1.0\"}"
  Subsystem3 : Subsystem
      settings: PortSchema="{\"entries\":[{\"content\":{\"sides\":[{\"content\":{\"connectorIds\":[\"In1\",\"In2\"]},\"type\":\"ConnectorPlacement.EquallySpacedRectSide\",\"uuid\":\"29da7ffb-f2b1-4a15-a75b-3bfe02cc4583\"},{\"content\":{\"connectorIds\":[\"Out1\"],\"side\":\"RIGHT\"},\"type\":\"ConnectorPlacement.EquallySpacedRectSide\",\"uuid\":\"eec62153-4e73-4349-8f3d-d93dc4ea66d4\"},{\"content\":{\"connectorIds\":[\"In3\"],\"side\":\"TOP\"},\"type\":\"ConnectorPlacement.EquallySpacedRectSide\",\"uuid\":\"568b9e49-e15d-457d-b854-c7ada7b8e177\"},{\"content\":{\"connectorIds\":[\"Out2\"],\"side\":\"BOTTOM\"},\"type\":\"ConnectorPlacement.EquallySpacedRectSide\",\"uuid\":\"d1e23110-4cf0-491e-9e49-dff7096ab241\"}]},\"type\":\"ConnectorPlacement.EquallySpacedConnector\",\"uuid\":\"de271efe-c0fb-43e0-95ac-ac6d3567011c\"}],\"packageUris\":[\"http://schema.mathworks.com/mf0/Connector/R2020b\"],\"version\":\"1.0\"}"
  To Workspace : ToWorkspace  VariableName=phase  SampleTime=Dt_var
  Phase number : Outport
  off_PH1.1 : Outport  Port=2
  off_PH1.2 : Outport  Port=3
  off_PH2.1 : Outport  Port=4
  off_PH2.2 : Outport  Port=5
  wires:
  Gain/1 -> Max/5  "start FA"
  Multiply/1 -> Max/3  "start RB 1"
  Multiply1/1 -> Max/2  "start hohmann 2"
  Multiply2/1 -> Max/1  "start hohmann 1"
  Multiply3/1 -> Max/4  "start RB2"
  Subsystem/1(Out1) -> Multiply3/1
  Subsystem1/1(Out1) -> Multiply2/1
  Subsystem2/1(Out1) -> Multiply1/1
  Subsystem3/1(Out1) -> Multiply/1
  Subsystem1/2(off_PH1.1) -> off_PH1.1/1, Subsystem2/3(off_PH1.1)
  Subsystem2/2(off_PH1.2) -> off_PH1.2/1, Subsystem3/3(off_PH1.2)
  Subsystem3/2(off_PH2.1) -> off_PH2.1/1, Subsystem/3(off_PH2.1)
  Subsystem/2(off_PH2.2) -> Gain/1, off_PH2.2/1
  Pos/1 -> Subsystem1/1(Pos), Subsystem2/1(Pos), Subsystem/2(Pos), Subsystem3/1(x)
  Max/1 -> Phase number/1, To Workspace/1
  Vel/1 -> Subsystem/1(Vel), Subsystem1/2(Vel), Subsystem2/2(Vel), Subsystem3/2(Vel)

== system Simulink_6DoF_RV/POSITION/Position and Guidance ==
  Phase : Inport
  Pos : Inport  Port=2
  Vel : Inport  Port=3
  Add1 : Sum  Inputs=+++
  Final Approach : Subsystem  SystemSampleTime=0.02
  Free Drift : Subsystem  TreatAsAtomicUnit=on
  Hohmann : Subsystem  SystemSampleTime=1
  Radial Boost1 : Subsystem  SystemSampleTime=1
  Rate Transition : RateTransition  OutPortSampleTime=1
  Rate Transition1 : RateTransition  OutPortSampleTime=0.02
  Sum : Sum
  Fc : Outport
  wires:
  Radial Boost1/1(Fz_PH2) -> Add1/3
  Vel/1 -> Final Approach/3(Vel), Radial Boost1/3(Vel)
  Phase/1 -> Final Approach/1(Phase), Radial Boost1/1(Phase), Hohmann/1(Phase)
  Pos/1 -> Final Approach/2(Pos), Radial Boost1/2(Pos)
  Hohmann/1(Fx_PH1) -> Add1/2
  Sum/1 -> Fc/1
  Free Drift/1(No Force) -> Add1/1
  Add1/1 -> Rate Transition/1
  Rate Transition/1 -> Sum/1
  Rate Transition1/1 -> Sum/2
  Final Approach/1(Fc) -> Rate Transition1/1

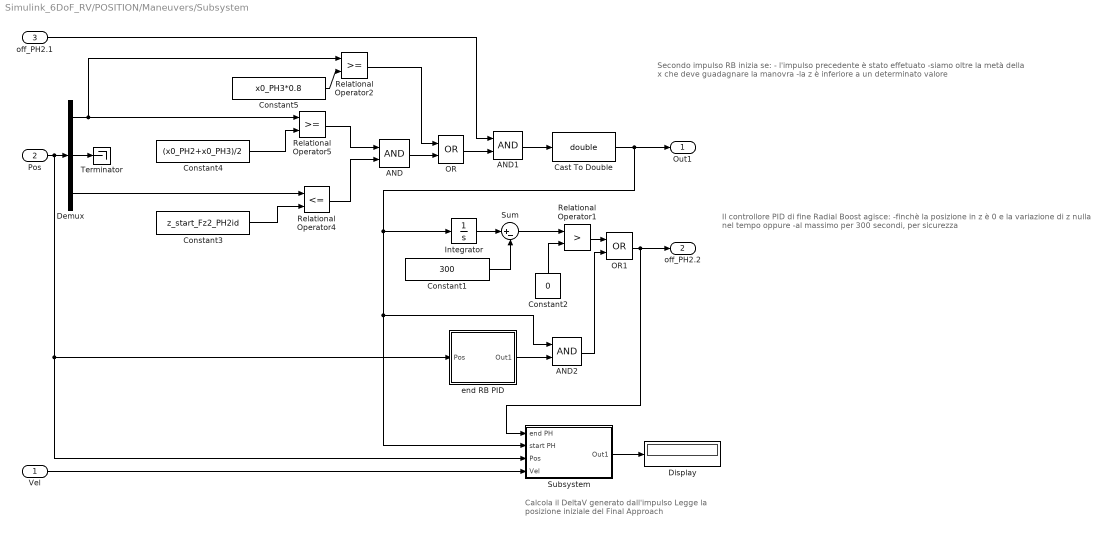
== system Simulink_6DoF_RV/POSITION/Maneuvers/Subsystem ==
  note: Calcola il DeltaV generato dall'impulso
      | Legge la posizione iniziale del Final Approach
  note: Il controllore PID di fine Radial Boost agisce:
      | -finchè la posizione in z è 0 e la variazione di z nulla nel tempo
      | oppure
      | -al massimo per 300 secondi, per sicurezza
  note: Secondo impulso RB inizia se:
      | - l'impulso precedente è stato effetuato
      | -siamo oltre la metà della x che deve guadagnare la manovra
      | -la z è inferiore a un determinato valore
  Vel : Inport
  Pos : Inport  Port=2
  off_PH2.1 : Inport  Port=3
  AND : Logic  AllPortsSameDT=off  OutDataTypeStr=boolean
  AND1 : Logic  AllPortsSameDT=off  OutDataTypeStr=boolean
  AND2 : Logic  AllPortsSameDT=off  OutDataTypeStr=boolean
  Cast To Double : DataTypeConversion  OutDataTypeStr=double
  Constant1 : Constant  Value=300
  Constant2 : Constant  Value=0
  Constant3 : Constant  Value=z_start_Fz2_PH2id
  Constant4 : Constant  Value=(x0_PH2+x0_PH3)/2
  Constant5 : Constant  Value=x0_PH3*0.8
  Demux : Demux  Outputs=3
  Display : Display
  Integrator : Integrator
  OR : Logic  Operator=OR  AllPortsSameDT=off  OutDataTypeStr=boolean
  OR1 : Logic  Operator=OR  AllPortsSameDT=off  OutDataTypeStr=boolean
  Relational Operator1 : RelationalOperator  Operator=>  OutDataTypeStr=boolean  RndMeth=Simplest
  Relational Operator2 : RelationalOperator  OutDataTypeStr=boolean  RndMeth=Simplest
  Relational Operator4 : RelationalOperator  Operator=<=  OutDataTypeStr=boolean  RndMeth=Simplest
  Relational Operator5 : RelationalOperator  OutDataTypeStr=boolean  RndMeth=Simplest
  Subsystem : Subsystem
  Sum : Sum  Inputs=|+-
  Terminator : Terminator
  end RB PID : Subsystem
  Out1 : Outport
  off_PH2.2 : Outport  Port=2
  wires:
  Constant4/1 -> Relational Operator5/2
  Constant3/1 -> Relational Operator4/2
  Relational Operator4/1 -> AND/2
  Relational Operator5/1 -> AND/1
  off_PH2.1/1 -> AND1/1
  Cast To Double/1 -> Out1/1, AND2/1, Subsystem/2(start PH), Integrator/1
  Sum/1 -> Relational Operator1/1
  Constant2/1 -> Relational Operator1/2
  Constant1/1 -> Sum/2
  Integrator/1 -> Sum/1
  Demux/2 -> Terminator/1
  Demux/3 -> Relational Operator4/1
  Vel/1 -> Subsystem/4(Vel)
  Subsystem/1(Out1) -> Display/1
  Demux/1 -> Relational Operator2/1, Relational Operator5/1
  Constant5/1 -> Relational Operator2/2
  AND/1 -> OR/2
  Relational Operator2/1 -> OR/1
  AND1/1 -> Cast To Double/1
  OR/1 -> AND1/2
  Relational Operator1/1 -> OR1/1
  OR1/1 -> off_PH2.2/1, Subsystem/1(end PH)
  Pos/1 -> end RB PID/1(Pos), Subsystem/3(Pos), Demux/1
  end RB PID/1(Out1) -> AND2/2
  AND2/1 -> OR1/2

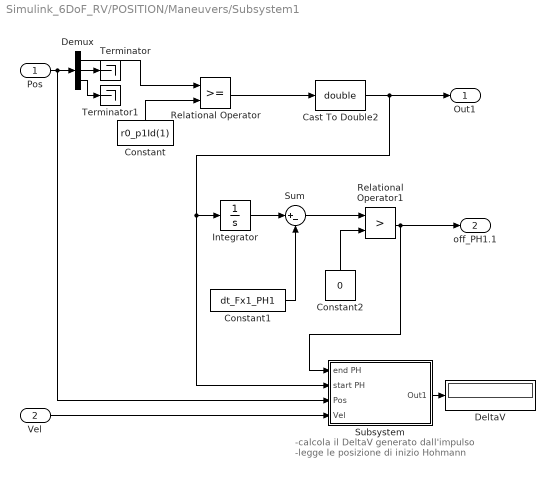
== system Simulink_6DoF_RV/POSITION/Maneuvers/Subsystem1 ==
  note: -calcola il DeltaV generato dall'impulso
      | -legge le posizione di inizio Hohmann
  Pos : Inport
  Vel : Inport  Port=2
  Cast To Double2 : DataTypeConversion  OutDataTypeStr=double
  Constant : Constant  Value=r0_p1Id(1)
  Constant1 : Constant  Value=dt_Fx1_PH1
  Constant2 : Constant  Value=0
  DeltaV : Display
  Demux : Demux  Outputs=3
  Integrator : Integrator
  Relational Operator : RelationalOperator  OutDataTypeStr=boolean  RndMeth=Simplest
  Relational Operator1 : RelationalOperator  Operator=>  OutDataTypeStr=boolean  RndMeth=Simplest
  Subsystem : Subsystem
  Sum : Sum  Inputs=|+-
  Terminator : Terminator
  Terminator1 : Terminator
  Out1 : Outport
  off_PH1.1 : Outport  Port=2
  wires:
  Constant/1 -> Relational Operator/2
  Cast To Double2/1 -> Out1/1, Subsystem/2(start PH), Integrator/1
  Relational Operator/1 -> Cast To Double2/1
  Integrator/1 -> Sum/1
  Sum/1 -> Relational Operator1/1
  Constant2/1 -> Relational Operator1/2
  Constant1/1 -> Sum/2
  Pos/1 -> Subsystem/3(Pos), Demux/1
  Demux/1 -> Relational Operator/1
  Demux/2 -> Terminator/1
  Demux/3 -> Terminator1/1
  Relational Operator1/1 -> off_PH1.1/1, Subsystem/1(end PH)
  Vel/1 -> Subsystem/4(Vel)
  Subsystem/1(Out1) -> DeltaV/1

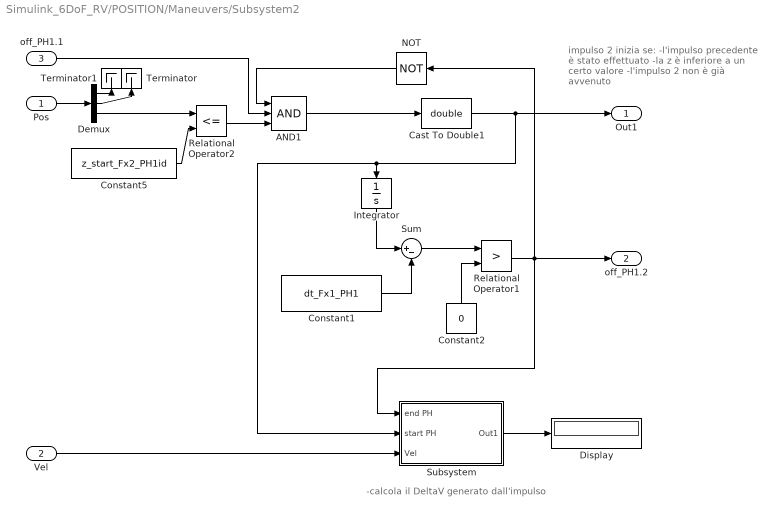
== system Simulink_6DoF_RV/POSITION/Maneuvers/Subsystem2 ==
  note: impulso 2 inizia se:
      | -l'impulso precedente è stato effettuato
      | -la z è inferiore a un certo valore
      | -l'impulso 2 non è già avvenuto
  note: -calcola il DeltaV generato dall'impulso
  Pos : Inport
  Vel : Inport  Port=2
  off_PH1.1 : Inport  Port=3
  AND1 : Logic  Inputs=3  AllPortsSameDT=off  OutDataTypeStr=boolean
  Cast To Double1 : DataTypeConversion  OutDataTypeStr=double
  Constant1 : Constant  Value=dt_Fx1_PH1
  Constant2 : Constant  Value=0
  Constant5 : Constant  Value=z_start_Fx2_PH1id
  Demux : Demux  Outputs=3
  Display : Display
  Integrator : Integrator
  NOT : Logic  Operator=NOT  IconShape=distinctive  AllPortsSameDT=off  OutDataTypeStr=boolean
  Relational Operator1 : RelationalOperator  Operator=>  OutDataTypeStr=boolean  RndMeth=Simplest
  Relational Operator2 : RelationalOperator  Operator=<=  OutDataTypeStr=boolean  RndMeth=Simplest
  Subsystem : Subsystem
  Sum : Sum  Inputs=|+-
  Terminator : Terminator
  Terminator1 : Terminator
  Out1 : Outport
  off_PH1.2 : Outport  Port=2
  wires:
  Constant5/1 -> Relational Operator2/2
  Relational Operator2/1 -> AND1/3
  off_PH1.1/1 -> AND1/2
  Integrator/1 -> Sum/1
  Sum/1 -> Relational Operator1/1
  Constant2/1 -> Relational Operator1/2
  Constant1/1 -> Sum/2
  Demux/3 -> Relational Operator2/1
  Pos/1 -> Demux/1
  Demux/2 -> Terminator/1
  Demux/1 -> Terminator1/1
  Vel/1 -> Subsystem/3(Vel)
  Subsystem/1(Out1) -> Display/1
  NOT/1 -> AND1/1
  Relational Operator1/1 -> off_PH1.2/1, NOT/1, Subsystem/1(end PH)
  AND1/1 -> Cast To Double1/1
  Cast To Double1/1 -> Subsystem/2(start PH), Integrator/1, Out1/1

== system Simulink_6DoF_RV/POSITION/Maneuvers/Subsystem3 ==
  note: Radial boost inizia appena è finito il secondo impulso della Hohmann
  note: -calcola il DeltaV generato dall'impulso
      | -legge le posizione di inizio Radial Boost
  x : Inport
  Vel : Inport  Port=2
  off_PH1.2 : Inport  Port=3
  Cast To Double : DataTypeConversion  OutDataTypeStr=double
  Constant4 : Constant  Value=0
  Display : Display
  Integrator : Integrator
  Relational Operator2 : RelationalOperator  Operator=>  OutDataTypeStr=boolean  RndMeth=Simplest
  Subsystem : Subsystem
  Sum1 : Sum  Inputs=|+-
  fire-time calculator : Subsystem  TreatAsAtomicUnit=on
  Out1 : Outport
  off_PH2.1 : Outport  Port=2
  wires:
  Cast To Double/1 -> Integrator/1, Out1/1
  Relational Operator2/1 -> Subsystem/1(end PH), off_PH2.1/1
  Sum1/1 -> Relational Operator2/1
  Constant4/1 -> Relational Operator2/2
  Integrator/1 -> Sum1/1
  fire-time calculator/1(dt_PH2_1) -> Sum1/2
  off_PH1.2/1 -> fire-time calculator/Trigger, Subsystem/2(off_PH1.2), Cast To Double/1
  Vel/1 -> fire-time calculator/2(Vel), Subsystem/4(Vel)
  Subsystem/1(Vz_final) -> Display/1
  x/1 -> fire-time calculator/1(x), Subsystem/3(x)

== system Simulink_6DoF_RV/POSITION/Position and Guidance/Final Approach ==
  Phase : Inport
  Pos : Inport  Port=2
  Vel : Inport  Port=3
  Bus Selector : BusSelector  OutputSignals=phase number
  If2 : If  IfExpression=u1==3  ShowElse=off
  Switch Case Action Subsystem : Subsystem  TreatAsAtomicUnit=on
  Fc : Outport
  wires:
  Pos/1 -> Switch Case Action Subsystem/1(Pos)
  Vel/1 -> Switch Case Action Subsystem/2(Vel)
  If2/1 -> Switch Case Action Subsystem/Action
  Switch Case Action Subsystem/1(Fc) -> Fc/1
  Phase/1 -> Bus Selector/1
  Bus Selector/1 -> If2/1  "<phase number>"

== system Simulink_6DoF_RV/POSITION/Position and Guidance/Free Drift ==
  Constant : Constant  Value=[0 0 0]'
  No Force : Outport
  wires:
  Constant/1 -> No Force/1

== system Simulink_6DoF_RV/POSITION/Position and Guidance/Hohmann ==
  Phase : Inport
  HN 1st & 2nd impulse : Subsystem  TreatAsAtomicUnit=on
  If : If  IfExpression=u1 == 1
  If Action Subsystem2 : Subsystem  TreatAsAtomicUnit=on
  Merge : Merge
  Subsystem : Subsystem
  Fx_PH1 : Outport
  wires:
  If/1 -> HN 1st & 2nd impulse/Action
  HN 1st & 2nd impulse/1(Fc_H1) -> Merge/1
  Phase/1 -> Subsystem/1(In1)
  Subsystem/1(fire_PH1) -> If/1
  If/2 -> If Action Subsystem2/Action
  If Action Subsystem2/1(F=0) -> Merge/2
  Merge/1 -> Fx_PH1/1

== system Simulink_6DoF_RV/POSITION/Position and Guidance/Radial Boost1 ==
  Phase : Inport
  Pos : Inport  Port=2
  Vel : Inport  Port=3
  " RB 2nd impulse control" : Subsystem  TreatAsAtomicUnit=on
  If : If  NumInputs=2  IfExpression=u1 == 1  ElseIfExpressions=u2==1
  If Action Subsystem2 : Subsystem  TreatAsAtomicUnit=on
  Merge : Merge  Inputs=3
  RB 1st impulse : Subsystem  TreatAsAtomicUnit=on
  Subsystem : Subsystem
  Fz_PH2 : Outport
  wires:
  If/2 -> " RB 2nd impulse control"/Action
  RB 1st impulse/1(Fc_H1) -> Merge/1
  Merge/1 -> Fz_PH2/1
  Subsystem/2(fire_PH2.2) -> If/2
  If/1 -> RB 1st impulse/Action
  Subsystem/1(fire_PH2.1) -> If/1
  Phase/1 -> Subsystem/1(In1)
  Vel/1 -> " RB 2nd impulse control"/2(Vel)
  Pos/1 -> " RB 2nd impulse control"/1(Pos)
  If/3 -> If Action Subsystem2/Action
  If Action Subsystem2/1(F=0) -> Merge/3
  " RB 2nd impulse control"/1(Fx) -> Merge/2

== system Simulink_6DoF_RV/POSITION/Maneuvers/Subsystem/Subsystem ==
  end PH : Inport
  start PH : Inport  Port=2
  Pos : Inport  Port=3
  Vel : Inport  Port=4
  Demux1 : Demux  Outputs=3
  Sum1 : Sum  Inputs=-+
  Terminator2 : Terminator
  Terminator3 : Terminator
  To Workspace : ToWorkspace  VariableName=pos_start_FA  SampleTime=Dt_var
  Triggered Subsystem1 : Subsystem  TreatAsAtomicUnit=on
  Triggered Subsystem2 : Subsystem  TreatAsAtomicUnit=on
  Out1 : Outport
  wires:
  Triggered Subsystem2/1(V_in) -> Sum1/1
  Triggered Subsystem1/1(V_fin) -> Sum1/2
  Vel/1 -> Triggered Subsystem2/1(Vel), Triggered Subsystem1/1(Vel)
  end PH/1 -> Triggered Subsystem1/Trigger
  start PH/1 -> Triggered Subsystem2/Trigger
  Demux1/3 -> Out1/1
  Sum1/1 -> Demux1/1
  Demux1/1 -> Terminator2/1
  Demux1/2 -> Terminator3/1
  Pos/1 -> Triggered Subsystem1/2(Pos)
  Triggered Subsystem1/2(start_FA) -> To Workspace/1

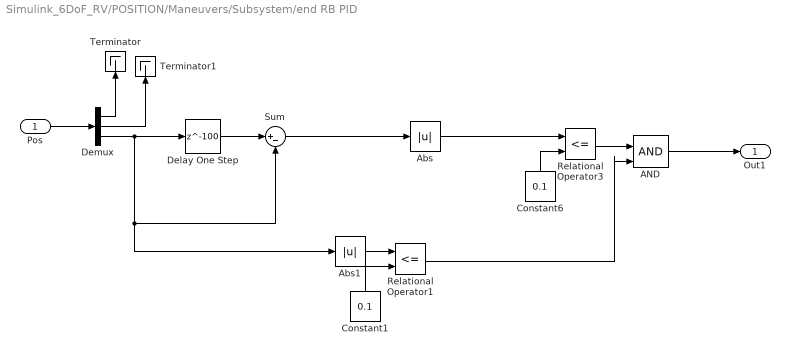
== system Simulink_6DoF_RV/POSITION/Maneuvers/Subsystem/end RB PID ==
  Pos : Inport
  AND : Logic  IconShape=distinctive  AllPortsSameDT=off  OutDataTypeStr=boolean
  Abs : Abs
  Abs1 : Abs
  Constant1 : Constant  Value=0.1
  Constant6 : Constant  Value=0.1
  Delay One Step : Delay  DelayLength=100
  Demux : Demux  Outputs=3
  Relational Operator1 : RelationalOperator  Operator=<=  OutDataTypeStr=boolean  RndMeth=Simplest
  Relational Operator3 : RelationalOperator  Operator=<=  OutDataTypeStr=boolean  RndMeth=Simplest
  Sum : Sum  Inputs=|+-
  Terminator : Terminator
  Terminator1 : Terminator
  Out1 : Outport
  wires:
  Delay One Step/1 -> Sum/1
  Constant6/1 -> Relational Operator3/2
  Sum/1 -> Abs/1
  Abs/1 -> Relational Operator3/1
  Pos/1 -> Demux/1
  Demux/1 -> Terminator/1
  Demux/2 -> Terminator1/1
  Relational Operator3/1 -> AND/1
  AND/1 -> Out1/1
  Relational Operator1/1 -> AND/2
  Demux/3 -> Sum/2, Abs1/1, Delay One Step/1
  Constant1/1 -> Relational Operator1/2
  Abs1/1 -> Relational Operator1/1

== system Simulink_6DoF_RV/POSITION/Maneuvers/Subsystem1/Subsystem ==
  end PH : Inport
  start PH : Inport  Port=2
  Pos : Inport  Port=3
  Vel : Inport  Port=4
  Demux1 : Demux  Outputs=3
  Sum1 : Sum  Inputs=-+
  Terminator2 : Terminator
  Terminator3 : Terminator
  To Workspace : ToWorkspace  VariableName=pos_start_HN  SampleTime=Dt_var
  Triggered Subsystem1 : Subsystem  TreatAsAtomicUnit=on
  Triggered Subsystem2 : Subsystem  TreatAsAtomicUnit=on
  Out1 : Outport
  wires:
  Triggered Subsystem2/1(V_in) -> Sum1/1
  Triggered Subsystem1/1(V_fin) -> Sum1/2
  Sum1/1 -> Demux1/1
  Vel/1 -> Triggered Subsystem2/2(Vel), Triggered Subsystem1/1(Vel)
  Demux1/3 -> Terminator2/1
  Demux1/2 -> Terminator3/1
  end PH/1 -> Triggered Subsystem1/Trigger
  Demux1/1 -> Out1/1
  start PH/1 -> Triggered Subsystem2/Trigger
  Pos/1 -> Triggered Subsystem2/1(Pos)
  Triggered Subsystem2/2(Pos_HN_start) -> To Workspace/1

== system Simulink_6DoF_RV/POSITION/Maneuvers/Subsystem2/Subsystem ==
  end PH : Inport
  start PH : Inport  Port=2
  Vel : Inport  Port=3
  Demux1 : Demux  Outputs=3
  Sum1 : Sum  Inputs=-+
  Terminator2 : Terminator
  Terminator3 : Terminator
  Triggered Subsystem1 : Subsystem  TreatAsAtomicUnit=on
  Triggered Subsystem2 : Subsystem  TreatAsAtomicUnit=on
  Out1 : Outport
  wires:
  Triggered Subsystem2/1(V_in) -> Sum1/1
  Triggered Subsystem1/1(V_fin) -> Sum1/2
  Sum1/1 -> Demux1/1
  Vel/1 -> Triggered Subsystem2/1(Vel), Triggered Subsystem1/1(Vel)
  Demux1/3 -> Terminator2/1
  Demux1/2 -> Terminator3/1
  Demux1/1 -> Out1/1
  end PH/1 -> Triggered Subsystem1/Trigger
  start PH/1 -> Triggered Subsystem2/Trigger

== system Simulink_6DoF_RV/POSITION/Maneuvers/Subsystem3/Subsystem ==
  end PH : Inport
  off_PH1.2 : Inport  Port=2
  x : Inport  Port=3
  Vel : Inport  Port=4
  Demux2 : Demux  Outputs=3
  Terminator1 : Terminator
  Terminator4 : Terminator
  To Workspace : ToWorkspace  VariableName=pos_start_RB  SampleTime=Dt_var
  Triggered Subsystem1 : Subsystem  TreatAsAtomicUnit=on
  Triggered Subsystem3 : Subsystem  TreatAsAtomicUnit=on
  Vz_final : Outport
  wires:
  Vel/1 -> Triggered Subsystem1/1(Vel)
  end PH/1 -> Triggered Subsystem1/Trigger
  Demux2/3 -> Vz_final/1
  Triggered Subsystem1/1(V_fin) -> Demux2/1
  Demux2/1 -> Terminator1/1
  Demux2/2 -> Terminator4/1
  Triggered Subsystem3/1(Pos_RB_start) -> To Workspace/1
  x/1 -> Triggered Subsystem3/1(Pos)
  off_PH1.2/1 -> Triggered Subsystem3/Trigger

== system Simulink_6DoF_RV/POSITION/Maneuvers/Subsystem3/fire-time calculator ==
  x : Inport
  Vel : Inport  Port=2
  Trigger : TriggerPort  VariantControl=(inherit)
  Constant : Constant  Value=[mc, omega, Fz_PH2id, r0_p3Id(1),dtz_PH2_corr]
  MATLAB Function : MATLAB Function  TreatAsAtomicUnit=on
  dt_PH2_1 : Outport
  wires:
  Vel/1 -> MATLAB Function/1(Vel)
  Constant/1 -> MATLAB Function/3(data)
  MATLAB Function/1(dt_PH2_1) -> dt_PH2_1/1
  x/1 -> MATLAB Function/2(Pos)

== system Simulink_6DoF_RV/POSITION/Position and Guidance/Final Approach/Switch Case Action Subsystem ==
  Pos : Inport
  Vel : Inport  Port=2
  Action Port : ActionPort  ActionPortLabel=if(u1==3)
  Constant : Constant  Value=fa_control
  FA SMC : Subsystem  TreatAsAtomicUnit=on
  FA straight line : Subsystem  TreatAsAtomicUnit=on
  Merge : Merge
  Switch Case : SwitchCase  CaseConditions={1,2}  ShowDefaultCase=off
  Fc : Outport
  wires:
  Switch Case/2 -> FA SMC/Action
  Switch Case/1 -> FA straight line/Action
  Constant/1 -> Switch Case/1
  Pos/1 -> FA straight line/1(Pos), FA SMC/1(Pos)
  FA SMC/1(Fc) -> Merge/2
  FA straight line/1(Fc) -> Merge/1
  Vel/1 -> FA straight line/2(Vel), FA SMC/2(Vel)
  Merge/1 -> Fc/1

== system Simulink_6DoF_RV/POSITION/Position and Guidance/Hohmann/HN 1st & 2nd impulse ==
  Action Port : ActionPort  ActionPortLabel=if(u1 == 1)
  Constant : Constant  Value=[Fx_PH1id 0 0]'
  IC : InitialCondition  Value=[0 0 0]
  Fc_H1 : Outport
  wires:
  Constant/1 -> IC/1
  IC/1 -> Fc_H1/1

== system Simulink_6DoF_RV/POSITION/Position and Guidance/Hohmann/If Action Subsystem2 ==
  Action Port : ActionPort  ActionPortLabel=else
  Constant : Constant  Value=[0 0 0]'
  IC : InitialCondition  Value=[0 0 0]
  F=0 : Outport
  wires:
  Constant/1 -> IC/1
  IC/1 -> F=0/1

== system Simulink_6DoF_RV/POSITION/Position and Guidance/Hohmann/Subsystem ==
  In1 : Inport
  AND : Logic  AllPortsSameDT=off  OutDataTypeStr=boolean
  AND1 : Logic  AllPortsSameDT=off  OutDataTypeStr=boolean
  Bus Selector : BusSelector  OutputSignals=off_PH1:1,phase number,off_PH1:2
  Constant : Constant
  Constant1 : Constant  Value=1.5
  Equal : RelationalOperator  Operator===  OutDataTypeStr=boolean  RndMeth=Simplest
  Equal1 : RelationalOperator  Operator===  OutDataTypeStr=boolean  RndMeth=Simplest
  NOT : Logic  Operator=NOT  AllPortsSameDT=off  OutDataTypeStr=boolean
  NOT1 : Logic  Operator=NOT  AllPortsSameDT=off  OutDataTypeStr=boolean
  OR : Logic  Operator=OR  AllPortsSameDT=off  OutDataTypeStr=boolean
  fire_PH1 : Outport
  wires:
  Bus Selector/3 -> NOT1/1  "<off_PH1:2>"
  Bus Selector/1 -> NOT/1  "<off_PH1:1>"
  In1/1 -> Bus Selector/1
  Bus Selector/2 -> Equal/2, Equal1/1  "<phase number>"
  Constant/1 -> Equal/1
  Equal/1 -> AND/2
  AND/1 -> OR/1
  Constant1/1 -> Equal1/2
  NOT/1 -> AND/1
  Equal1/1 -> AND1/1
  NOT1/1 -> AND1/2
  AND1/1 -> OR/2
  OR/1 -> fire_PH1/1

== system Simulink_6DoF_RV/POSITION/Position and Guidance/Radial Boost1/ RB 2nd impulse control ==
  Pos : Inport
  Vel : Inport  Port=2
  Action Port : ActionPort  ActionPortLabel=elseif(u2==1)
  Pos z y : Subsystem
  Scope : Scope
  Sum2 : Sum
  Vel x : Subsystem
  Fx : Outport
  wires:
  Vel/1 -> Pos z y/2(In2), Vel x/1(In1)
  Sum2/1 -> Scope/1, Fx/1
  Vel x/1(Out1) -> Sum2/2
  Pos/1 -> Pos z y/1(In1)
  Pos z y/1(Out1) -> Sum2/1

== system Simulink_6DoF_RV/POSITION/Position and Guidance/Radial Boost1/If Action Subsystem2 ==
  Action Port : ActionPort  ActionPortLabel=else
  Constant : Constant  Value=[0 0 0]'
  IC : InitialCondition  Value=[0 0 0]
  F=0 : Outport
  wires:
  Constant/1 -> IC/1
  IC/1 -> F=0/1

== system Simulink_6DoF_RV/POSITION/Position and Guidance/Radial Boost1/RB 1st impulse ==
  Action Port : ActionPort  ActionPortLabel=if(u1 == 1)
  Constant : Constant  Value=[0 0 Fz_PH2id]'
  Fc_H1 : Outport
  wires:
  Constant/1 -> Fc_H1/1

== system Simulink_6DoF_RV/POSITION/Position and Guidance/Radial Boost1/Subsystem ==
  In1 : Inport
  AND : Logic  AllPortsSameDT=off  OutDataTypeStr=boolean
  AND1 : Logic  AllPortsSameDT=off  OutDataTypeStr=boolean
  Bus Selector : BusSelector  OutputSignals=off_PH2:1,phase number,off_PH2:2
  Constant : Constant  Value=2
  Constant1 : Constant  Value=2.5
  Equal : RelationalOperator  Operator===  OutDataTypeStr=boolean  RndMeth=Simplest
  Equal1 : RelationalOperator  Operator===  OutDataTypeStr=boolean  RndMeth=Simplest
  NOT : Logic  Operator=NOT  AllPortsSameDT=off  OutDataTypeStr=boolean
  NOT1 : Logic  Operator=NOT  AllPortsSameDT=off  OutDataTypeStr=boolean
  fire_PH2.1 : Outport
  fire_PH2.2 : Outport  Port=2
  wires:
  AND/1 -> fire_PH2.1/1
  AND1/1 -> fire_PH2.2/1
  NOT1/1 -> AND1/2
  Equal1/1 -> AND1/1
  NOT/1 -> AND/1
  Constant1/1 -> Equal1/2
  Equal/1 -> AND/2
  Constant/1 -> Equal/1
  Bus Selector/2 -> Equal1/1, Equal/2  "<phase number>"
  In1/1 -> Bus Selector/1
  Bus Selector/1 -> NOT/1  "<off_PH2:1>"
  Bus Selector/3 -> NOT1/1  "<off_PH2:2>"

== system Simulink_6DoF_RV/POSITION/Maneuvers/Subsystem/Subsystem/Triggered Subsystem1 ==
  Vel : Inport
  Pos : Inport  Port=2
  Trigger : TriggerPort  VariantControl=(inherit)
  V_fin : Outport
  start_FA : Outport  Port=2
  wires:
  Vel/1 -> V_fin/1
  Pos/1 -> start_FA/1

== system Simulink_6DoF_RV/POSITION/Maneuvers/Subsystem/Subsystem/Triggered Subsystem2 ==
  Vel : Inport
  Trigger : TriggerPort  VariantControl=(inherit)
  V_in : Outport
  wires:
  Vel/1 -> V_in/1

== system Simulink_6DoF_RV/POSITION/Maneuvers/Subsystem1/Subsystem/Triggered Subsystem1 ==
  Vel : Inport
  Trigger : TriggerPort  VariantControl=(inherit)
  V_fin : Outport
  wires:
  Vel/1 -> V_fin/1

== system Simulink_6DoF_RV/POSITION/Maneuvers/Subsystem1/Subsystem/Triggered Subsystem2 ==
  Pos : Inport
  Vel : Inport  Port=2
  Trigger : TriggerPort  VariantControl=(inherit)
  V_in : Outport
  Pos_HN_start : Outport  Port=2
  wires:
  Vel/1 -> V_in/1
  Pos/1 -> Pos_HN_start/1

== system Simulink_6DoF_RV/POSITION/Maneuvers/Subsystem2/Subsystem/Triggered Subsystem1 ==
  Vel : Inport
  Trigger : TriggerPort  VariantControl=(inherit)
  V_fin : Outport
  wires:
  Vel/1 -> V_fin/1

== system Simulink_6DoF_RV/POSITION/Maneuvers/Subsystem2/Subsystem/Triggered Subsystem2 ==
  Vel : Inport
  Trigger : TriggerPort  VariantControl=(inherit)
  V_in : Outport
  wires:
  Vel/1 -> V_in/1

== system Simulink_6DoF_RV/POSITION/Maneuvers/Subsystem3/Subsystem/Triggered Subsystem1 ==
  Vel : Inport
  Trigger : TriggerPort  VariantControl=(inherit)
  V_fin : Outport
  wires:
  Vel/1 -> V_fin/1

== system Simulink_6DoF_RV/POSITION/Maneuvers/Subsystem3/Subsystem/Triggered Subsystem3 ==
  Pos : Inport
  Trigger : TriggerPort  VariantControl=(inherit)
  Pos_RB_start : Outport
  wires:
  Pos/1 -> Pos_RB_start/1

== system Simulink_6DoF_RV/POSITION/Position and Guidance/Final Approach/Switch Case Action Subsystem/FA SMC ==
  Pos : Inport
  Vel : Inport  Port=2
  Action Port : ActionPort  ActionPortLabel=case [ 2 ]:
  " " : Constant  Value=Vx_max
  Constant : Constant  Value=Tmax
  Constant1 : Constant  Value=[lambda_FA, epsilon_FA]
  Constant2 : Constant  Value=[omega,mc]
  MATLAB Function : MATLAB Function  TreatAsAtomicUnit=on
  Pos desiderata : Constant  Value=r_des_fa
  Scope : Scope
  Sum : Sum  Inputs=-+|
  Sum1 : Sum  Inputs=-+|
  Vel desiderata : Constant  Value=v_des_fa
  Fc : Outport
  wires:
  Constant/1 -> MATLAB Function/3(max)
  Constant1/1 -> MATLAB Function/4(ctrl_var)
  MATLAB Function/1(F) -> Scope/1, Fc/1
  Vel/1 -> Sum/2
  Sum1/1 -> MATLAB Function/2(Pos)
  Pos/1 -> Sum1/2
  Vel desiderata/1 -> Sum/1
  Pos desiderata/1 -> Sum1/1
  Sum/1 -> MATLAB Function/1(Vel)
  " "/1 -> MATLAB Function/5(Vx_max)
  Constant2/1 -> MATLAB Function/6(omega_mc)
